simulink library "ep5_lib"  (R2023b)
settings: Solver=VariableStepAuto  StartTime=0.0  StopTime=10.0  RelTol=1e-3
settings Model: Creator=86186  LastModifiedBy=86186

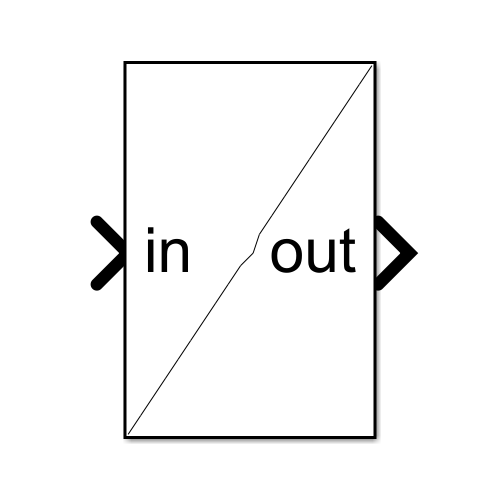
[thumbnail: Simulink's stored preview of the top-level diagram]
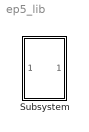
== system ep5_lib ==
  Subsystem : Subsystem  mask{a=3, b=4}
      mask init:
      | t = 0:0.1:2;
      | y = 3*t +4;
      mask DialogControl ParameterGroupVar Prompt: 参数
      mask Display:
      | plot(t,y);
      | port_label('input', 1, 'in');
      | port_label('output', 1, 'out');

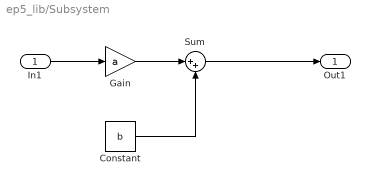
== system ep5_lib/Subsystem ==
  In1 : Inport
  Constant : Constant  Value=b
  Gain : Gain  Gain=a
  Sum : Sum  Inputs=|++
  Out1 : Outport
  wires:
  Constant/1 -> Sum/2
  Gain/1 -> Sum/1
  In1/1 -> Gain/1
  Sum/1 -> Out1/1
